simulink model "LADRC"  (R2025a)
settings: Solver=VariableStepAuto  StartTime=0  StopTime=10  FixedStep=0.001  RelTol=1e-5
InitFcn:
  | %wc=30;
  | %wo=290;
  | L1=3*wo;
  | L2=3*wo^2;
  | L3=wo^2;
  | Ke=50;
  | k1=wc^2;
  | k2=2*wc;
  | Rs=13.5;
  | Ms=0.05;
  | b=Ke/(Rs*Ms);
  | bs=0.008;
  | a=(1/Ms)*(bs+((Ke^2)/Rs));
model workspace (MAT data in the model file):
  Amp = 0.0011
values from neighbouring files (symbols this model uses):
  Ref = 0.001    [InitialParameter.m]
  wc = 95    [InitialParameter.m]    (also in pneumatic_code.m = 20.5)
settings Model: Creator=ply  LastModifiedBy=Steve
settings OptimizationCC: ZeroExternalMemoryAtStartup=off  ZeroInternalMemoryAtStartup=off
settings RTWCC: TargetLang=C++
settings GRTTargetCC: TargetLangStandard=C++11 (ISO)  CodeInterfacePackaging=C++ class

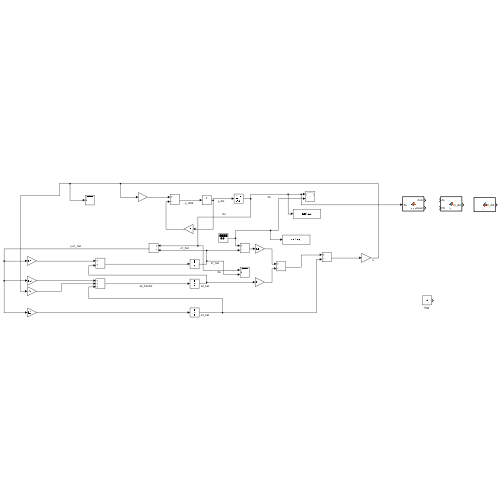
[thumbnail: Simulink's stored preview of the top-level diagram]
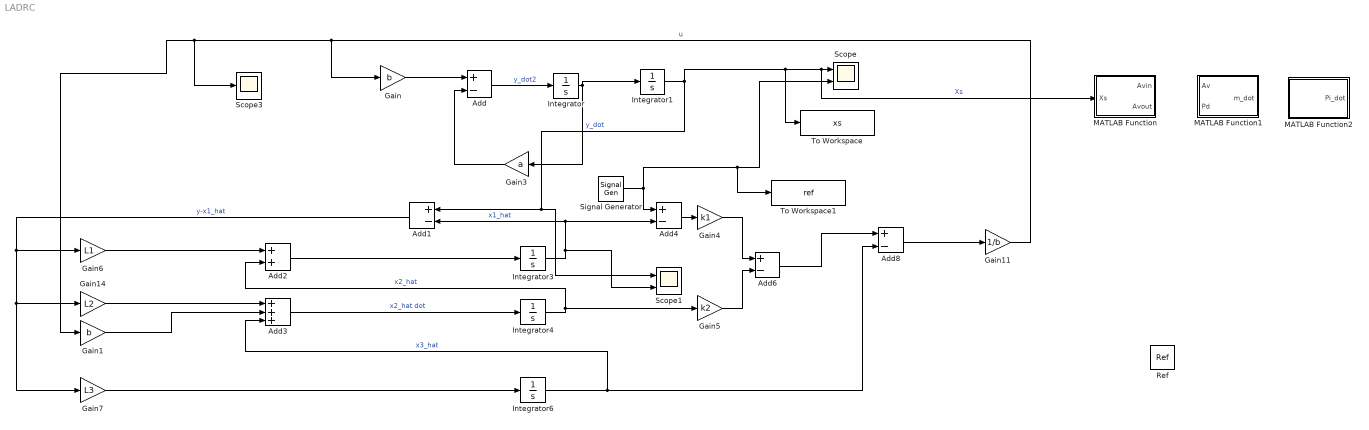
== system LADRC ==
  Add{,1,4,6,8} (5 alike) : Sum  Inputs=+-
  Add2 : Sum
  Add3 : Sum  Inputs=+++
  Gain : Gain  Gain=b
  Gain1 : Gain  Gain=b
  Gain11 : Gain  Gain=1/b
  Gain14 : Gain  Gain=L2
  Gain3 : Gain  Gain=a
  Gain4 : Gain  Gain=k1
  Gain5 : Gain  Gain=k2
  Gain6 : Gain  Gain=L1
  Gain7 : Gain  Gain=L3
  Integrator{,3..4,6} (4 alike) : Integrator
  Integrator1 : Integrator  LimitOutput=on  UpperSaturationLimit=0.0011  LowerSaturationLimit=-0.0011
  MATLAB Function : MATLAB Function  TreatAsAtomicUnit=on
  MATLAB Function1 : MATLAB Function  TreatAsAtomicUnit=on
  MATLAB Function2 : MATLAB Function  TreatAsAtomicUnit=on
  Ref : Constant  Value=Ref
  Scope : Scope  NumInputPorts=2
      settings: ActiveDisplayYMinimum=0.00081  ActiveDisplayYMaximum=0.00117
  Scope1 : Scope  NumInputPorts=2
      settings: ActiveDisplayYMinimum=-0.00138  ActiveDisplayYMaximum=0.00138
  Scope3 : Scope
      settings: ActiveDisplayYMinimum=-9.25803  ActiveDisplayYMaximum=9.25693  DataLoggingVariableName=ScopeData3
  Signal Generator : SignalGenerator  WaveForm=square  Amplitude=0.0011
  To Workspace : ToWorkspace  VariableName=xs  SaveFormat=Structure  SampleTime=-1
  To Workspace1 : ToWorkspace  VariableName=ref  SaveFormat=Structure  SampleTime=-1
  wires:
  Integrator/1 -> Integrator1/1, Gain3/1  "y_dot"
  Integrator1/1 -> Add1/1, Scope1/1, To Workspace/1, MATLAB Function/1(Xs), Scope/1  "Xs"
  Add/1 -> Integrator/1  "y_dot2"
  Gain/1 -> Add/1
  Gain3/1 -> Add/2
  Integrator3/1 -> Scope1/2, Add1/2, Add4/2  "x1_hat"
  Add2/1 -> Integrator3/1
  Integrator4/1 -> Gain5/1, Add2/2  "x2_hat"
  Add3/1 -> Integrator4/1  "x2_hat dot"
  Gain14/1 -> Add3/1
  Add1/1 -> Gain14/1, Gain7/1, Gain6/1  "y-x1_hat"
  Gain7/1 -> Integrator6/1
  Gain11/1 -> Gain/1, Scope3/1, Gain1/1  "u"
  Gain6/1 -> Add2/1
  Add4/1 -> Gain4/1
  Gain1/1 -> Add3/2
  Gain4/1 -> Add6/1
  Gain5/1 -> Add6/2
  Add6/1 -> Add8/1
  Integrator6/1 -> Add3/3, Add8/2  "x3_hat"
  Add8/1 -> Gain11/1
  Signal Generator/1 -> Add4/1, To Workspace1/1, Scope/2

== matlab function LADRC/MATLAB Function ==
  data: Xs input; Avin output; Avout output
function [Avin,Avout]= area(Xs)
nh = 4;
Pw = 0.0024;
Rh = 0.0019;
ph1 = 2*Rh^2*atan(sqrt((Rh-Pw+Xs)/(Rh+Pw-Xs)))-(Pw-Xs)*sqrt(Rh^2 - (Pw - Xs)^2);
ph2 = 2*Rh^2*atan(sqrt((Rh-Pw+abs(Xs))/(Rh+Pw-abs(Xs))))-(Pw-abs(Xs))*sqrt(Rh^2 - (Pw - abs(Xs))^2);
if Xs<=Pw-Rh
    Avin = 0;
elseif (Pw-Rh<Xs)&&(Xs<Pw+Rh)
    Avin = nh*ph1;
elseif Xs >= Pw+Rh
    Avin = pi*nh*Rh^2;
end

if Xs<=Pw-Rh
    Avout = pi*nh*Rh^2;
elseif (-Pw-Rh<Xs)&&(Xs<-Pw+Rh)
    Avout = nh*ph2;
elseif Xs >=-Pw+Rh
    Avout = 0;
end

end

== matlab function LADRC/MATLAB Function2 ==
  data: Pi_dot output
function Pi_dot = fcn()

y = u;

== matlab function LADRC/MATLAB Function1 ==
  data: Av input; m_dot output; Pd input
function m_dot = fcn(Av,Pd)
% C1 = sqrt(k/R*(2/(k+1)^((k+1)/(k-1))));
% C2 = sqrt(2*k/(R*(k-1)));
Pu = 758420;

C1 = 0.0404;
C2 = 0.1561;
Pcr = 0.528;
k = 1.4;
if (Pd/Pu)<Pcr
    m_dot = Cf*Av*C1*Pu/sqrt(T);
elseif (Pd/Pu)>Pcr
     m_dot = Cf*Av*C2*Pu/sqrt(T)*(Pd/Pu)^(1/k)*sqrt(1-((Pd/Pu)^((k-1)/k)));
end

end
